simulink model "SP_1a_sim"  (R2016a)
settings: Solver=VariableStepAuto  StartTime=0.0  StopTime=1000  RelTol=1e-3
settings Model: Creator=kuhaj  LastModifiedBy=Lukas Kolbl
settings DataIOCC: LimitDataPoints=on
settings DebuggingCC: AllowSymbolicDim=off
settings ModelReferenceCC: PropagateSignalLabelsOutOfModel=off
settings GRTTargetCC: GeneratePreprocessorConditionals=Use local settings

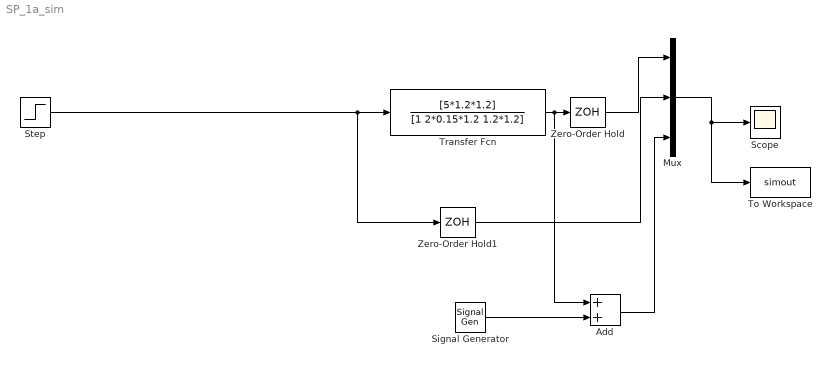
== system SP_1a_sim ==
  Add : Sum
  Mux : Mux  Inputs=3
  Scope : Scope
  Signal Generator : SignalGenerator  Units=rad/sec
  Step : Step  Time=0  SampleTime=0
  To Workspace : ToWorkspace  VariableName=simout  SaveFormat=Timeseries  SampleTime=-1
  Transfer Fcn : TransferFcn  Numerator=[5*1.2*1.2]  Denominator=[1 2*0.15*1.2 1.2*1.2]
  Zero-Order Hold : ZeroOrderHold  SampleTime=0.2
  Zero-Order Hold1 : ZeroOrderHold  SampleTime=0.2
  wires:
  Transfer Fcn/1 -> Add/1, Zero-Order Hold/1
  Mux/1 -> To Workspace/1, Scope/1
  Step/1 -> Zero-Order Hold1/1, Transfer Fcn/1
  Zero-Order Hold/1 -> Mux/1
  Zero-Order Hold1/1 -> Mux/2
  Signal Generator/1 -> Add/2
  Add/1 -> Mux/3
